simulink model "Fb_inverter3"  (Simulink 6.1)
settings: Solver=ode45  StartTime=0.0  StopTime=10.0  RelTol=1e-3
undefined symbols (not defined in the file): Ts
libraries: powerlib x8, powerlib_extras x1
settings Model: LastModifiedBy=ThinkPad
settings DebuggingCC: SolverPrmCheckMsg=warning

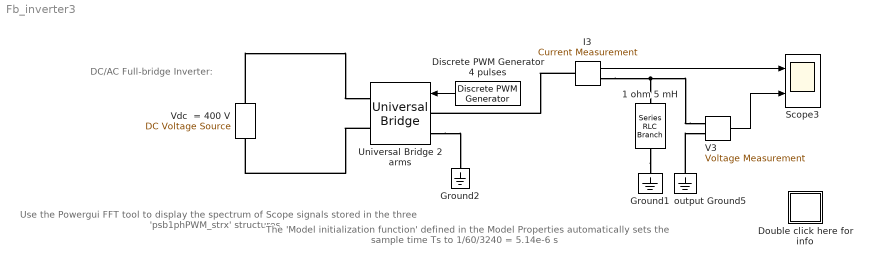
== system Fb_inverter3 ==
  note: Use the Powergui FFT tool to display the
      | spectrum of Scope  signals stored in the
      | three 'psb1phPWM_strx' structures
  note: DC/AC Full-bridge Inverter:
  note: The 'Model  initialization function' defined in the
      | Model Properties automatically sets the sample time Ts
      | to 1/60/3240 = 5.14e-6 s
  "1 ohm 5 mH " : powerlib/Elements/Series RLC Branch  Orientation=down  PhysicalDomain=powersysdomain  SubClassName=unknown  LeftPortType=p1  RightPortType=p1  LConnTagsString=__new0  RConnTagsString=__new0  Resistance=1  Inductance=5e-03  Capacitance=inf  Measurements=None
  Discrete PWM Generator 4 pulses : powerlib_extras/Discrete  Control Blocks/Discrete PWM Generator  Orientation=left  GeneratorMode="2-arm  bridge (4 pulses)"  Fc=1080  Ts=Ts  Internal=on  mIndex=0.8  Freq=60  Phase=0
  Double click here for info : Subsystem
      mask Display: disp('?')
  Ground1 : powerlib/Elements/Ground  Orientation=down  PhysicalDomain=powersysdomain  SubClassName=unknown  LeftPortType=p1  RightPortType=p1  LConnTagsString=a
  Ground2 : powerlib/Elements/Ground  Orientation=down  PhysicalDomain=powersysdomain  SubClassName=unknown  LeftPortType=p1  RightPortType=p1  LConnTagsString=a
  "I3 " : powerlib/Measurements/Current Measurement  Tag=PoWeRsYsTeMmEaSuReMeNt  PhasorSimulation=off  OutputType=Magnitude  PSBequivalent=0
  Scope3 : Scope  NumInputPorts=2
      settings: TimeRange=0.1  YMin=-200~-500  YMax=200~500  SaveName=psb1phPWM3_str  MaxDataPoints=500000
  Universal Bridge 2 arms : powerlib/Power Electronics/Universal Bridge  Orientation=left  Arms=2  SnubberResistance=10000  SnubberCapacitance=inf  Device=IGBT / Diodes  Ron=1e-4  Lon=0  ForwardVoltages="[  1  1  ]"  ForwardVoltage=.8  GTOparameters=[ 10e-6 , 20e-6 ]  IGBTparameters=[ 1e-6 , 2e-6 ]  Measurements=None
  V3 : powerlib/Measurements/Voltage Measurement  Tag=PoWeRsYsTeMmEaSuReMeNt  PhasorSimulation=off  OutputType=Magnitude  PSBequivalent=0
  "Vdc  = 400 V  " : powerlib/Electrical Sources/DC Voltage Source  Description=source block  Orientation=up  Amplitude=400  Measurements=None
      settings: AttributesFormatString=\n
  output Ground5 : powerlib/Elements/Ground  Orientation=down  PhysicalDomain=powersysdomain  SubClassName=unknown  LeftPortType=p1  RightPortType=p1  LConnTagsString=a
  wires:
  Discrete PWM Generator 4 pulses/1 -> Universal Bridge 2 arms/1
  "I3 "/1 -> Scope3/1
  V3/1 -> Scope3/2
  connections:
  V3/LConn1 -- "I3 "/RConn1 -- "1 ohm 5 mH "/LConn1
  "1 ohm 5 mH "/RConn1 -- Ground1/LConn1
  output Ground5/LConn1 -- V3/LConn2
  Universal Bridge 2 arms/RConn2 -- "Vdc  = 400 V  "/LConn1
  "Vdc  = 400 V  "/RConn1 -- Universal Bridge 2 arms/RConn1
  Universal Bridge 2 arms/LConn2 -- Ground2/LConn1
  "I3 "/LConn1 -- Universal Bridge 2 arms/LConn1

== system Fb_inverter3/Double click here for info ==
  note: G. Sybille and P. Giroux (Hydro-Quebec)
  note: Demonstration
  note: Circuit Description
  note: This demonstration illustrates use of the Universal Bridge and Discrete PWM Pulse Generator blocks
      | It also demonstrates harmonic analysis of PWM waveforms using the Powergui/FFT tool.
  note: The system consists of three independant circuits illustrating various PWM DC/DC and DC/AC inverters.
      | All converters are controlled in open loop with the Discrete PWM Generator block available in the Extras/Discrete Control Blocks library.
      | The three circuits use the same DC voltage (Vdc = 400V), carrier frequency (1080 Hz) and modulation index (m = 0.8) .
      | From top to bottom, the three circuits are:
      |
      | 1. DC/DC, two-quadrant converter (one-arm; two-switches)
      | 2. DC/AC,  half-bridge, bipolar converter  (one-arm; two-switches)
      | 3. DC/AC,  full-bridge, monopolar converter (two-arms; four-switches)
      |
      | In order to allow further signal processing, signals displayed on the three Scope blocks  (sampled at simulation sampling rate of 3240 samples/cycle)
      | are stored in three  variables named 'psb1phPWM1_str' , 'psb1phPWM2_str'  and  'psb1phPWM3_str'  (structures with time).
  note: Run the simulation and observe the following two waveforms on the three Scope blocks:
      | current into the load (trace 1), voltage generated by the PWM inverter (trace 2).
      |
      | Once the  simulation is completed, open the Powergui and select "FFT Analysis" to display the 0 - 5000 Hz frequency spectrum of signals saved
      | in the three "psb1phPWMx_str" structures. The FFT will be performed on  a 2-cycle window starting at t = 0.1 - 2/60 (last 2 cycles of recording).
      | For each circuit, selelect Input labeled "V inverter" . Click on "Display" and observe the frequency spectrum of last 2 cycles.
      |
      | The fundamental component of  V inverter (DC component in case of circuit 1) is displayed above the spectrum window.
      | Compare the magnitude of the fundamental or DC component of the inverter voltage with the theoretical values given in the  circuit.
      | Compare also the harmonic contents in the inverter voltage for the half-bridge and the full-bridge DC/AC inverters.
      |
      | The half-bridge inverter generates a bipolar voltage (-200V or +200V) .
      | Harmonics occur around the carrier frequency (1080 Hz +- k*60 Hz), with a maximum of 103% at 1080 Hz.
      |
      | The full-bridge inverter generates a monopolar voltage varying between 0 and+400V for one half cycle and then between 0 and -400V for the next half cycle.
      | For the same DC voltage and modulation index, the fundamental component magnitude is twice the value obtained with the half-bridge.
      | Harmonics generated by the full-bridge are lower and they appear at double of the carrier frequency (maximum of 40% at 2*1080+-60 Hz)
      |  As a result, the current obtained with the full-bridge is "cleaner".
      |
      | If you now perform a FFT on the signal "Iload" you will notice that the THD of load current is 7.3% for the half-bridge inverter as compared to
      | only  2% for the full-bridge inverter.
